simulink model "VelocityControl"  (R2024b)
settings: Solver=VariableStepAuto  StartTime=0.0  StopTime=60  RelTol=1e-3
undefined symbols (not defined in the file or in its folder): Kdu, Kdw, Kiu, Kiw, Kpu, Kpw
libraries: slpidlib x2
settings Model: Creator=Arghya  LastModifiedBy=Arghya

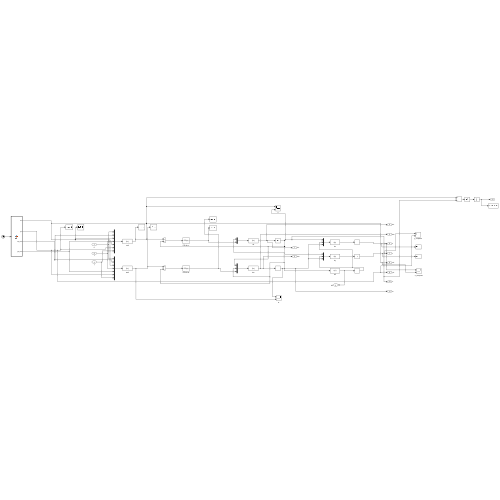
[thumbnail: Simulink's stored preview of the top-level diagram]
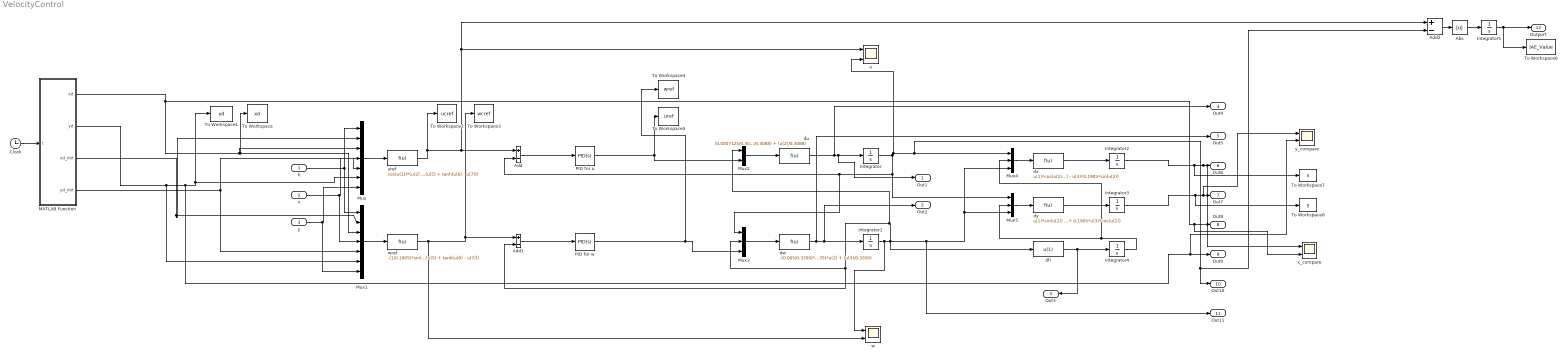
== system VelocityControl ==
  fi : Inport
  x : Inport  Port=2
  y : Inport  Port=3
  Abs : Abs  SaturateOnIntegerOverflow=off
  Add : Sum  Inputs=+-
  Add1 : Sum  Inputs=+-
  Add2 : Sum  Inputs=+-
  Clock : Clock
  Integrator : Integrator  ContinuousStateAttributes="\"u\""
  Integrator1 : Integrator  ContinuousStateAttributes="\"w\""
  Integrator{2..5} (4 alike) : Integrator
  MATLAB Function : MATLAB Function  TreatAsAtomicUnit=on
  Mux : Mux  Inputs=7
  Mux1 : Mux  Inputs=7
  Mux2 : Mux  Inputs=2
  Mux3 : Mux  Inputs=3
  Mux4 : Mux  Inputs=3
  Mux5 : Mux  Inputs=3
  PID for u : slpidlib/PID Controller  Controller=PID  Form=Parallel  TimeDomain=Continuous-time  UseExternalTs=off  SampleTime=-1  IntegratorMethod=Forward Euler  FilterMethod=Forward Euler  ControllerParametersSource=internal  P=Kpu  I=Kiu  UseKiTs=off  D=Kdu  UseExternalDerivativeSource=off  N=100  UseFilter=on  TunerSelectOption=Transfer Function Based (PID Tuner App)  InitialConditionSource=internal  InitialConditionForIntegrator=0  InitialConditionForFilter=0  DifferentiatorICPrevScaledInput=0  ExternalReset=none  TrackingMode=off  Kt=1  LimitOutput=off  SatLimitsSource=internal  UpperSaturationLimit=inf  LowerSaturationLimit=-inf  LinearizeAsGain=on  AntiWindupMode=none  Kb=1  LimitIntegrator=off  UpperIntegratorSaturationLimit=inf  LowerIntegratorSaturationLimit=-inf  POutMin=[]  POutMax=[]  IOutMin=[]  IOutMax=[]  DOutMin=[]  DOutMax=[]  NOutMin=[]  NOutMax=[]  SumOutMin=[]  SumOutMax=[]  SaturationOutMin=[]  SaturationOutMax=[]  PParamMin=[]  PParamMax=[]  IParamMin=[]  IParamMax=[]  DParamMin=[]  DParamMax=[]  NParamMin=[]  NParamMax=[]  KbParamMin=[]  KbParamMax=[]  KtParamMin=[]  KtParamMax=[]  KbOutMin=[]  KbOutMax=[]  KtOutMin=[]  KtOutMax=[]  IntegratorOutMin=[]  IntegratorOutMax=[]  FilterOutMin=[]  FilterOutMax=[]  SumI1OutMin=[]  SumI1OutMax=[]  SumI2OutMin=[]  SumI2OutMax=[]  SumI3OutMin=[]  SumI3OutMax=[]  SumI4OutMin=[]  SumI4OutMax=[]  SumDOutMin=[]  SumDOutMax=[]  DifferentiatorOutMin=[]  DifferentiatorOutMax=[]  FilterDiffOutCoefMin=[]  FilterDiffOutCoefMax=[]  ReciprocalOutMin=[]  ReciprocalOutMax=[]  SumDenOutMin=[]  SumDenOutMax=[]  SumNumOutMin=[]  SumNumOutMax=[]  DivideOutMin=[]  DivideOutMax=[]  UdiffTsProdOutMin=[]  UdiffTsProdOutMax=[]  NTsProdOutMin=[]  NTsProdOutMax=[]  UintegralTsProdOutMin=[]  UintegralTsProdOutMax=[]  UngainTsProdOutMin=[]  UngainTsProdOutMax=[]  ClampingZeroOutDataTypeStr=Inherit: Inherit via back propagation  ClampingZeroOutMin=[]  ClampingZeroOutMax=[]  FilterDenConstantOutDataTypeStr=Inherit: Inherit via back propagation  FilterDenConstantOutMin=[]  FilterDenConstantOutMax=[]  PCopyOutDataTypeStr=Inherit: Inherit via back propagation  PCopyOutMin=[]  PCopyOutMax=[]  NCopyOutDataTypeStr=Inherit: Inherit via back propagation  NCopyOutMin=[]  NCopyOutMax=[]  IntegratorContinuousStateAttributes=''  IntegratorStateMustResolveToSignalObject=off  IntegratorRTWStateStorageClass=Auto  FilterContinuousStateAttributes=''  FilterStateMustResolveToSignalObject=off  FilterRTWStateStorageClass=Auto  ParallelPVariant=InternalParameters  IdealPVariant=Disabled  IVariant=InternalParameters  DVariant=InternalParameters  IntegratorVariant=Continuous  SatVariant=Disabled  AWVariant=Passthrough  PCopyVariant=Disabled  TRVariant=Disabled  FdbkBlocksVariant=Forward  IdealPFdbkVariant=Disabled  SatFdbkVariant=Disabled  DerivativeFilterVariant=ContFilter  NVariant=InternalParameters  NCopyVariant=Disabled  FilterICVariant=InternalICsFilter  IntegratorICVariant=InternalICs  ExternalResetVariant=Disabled  TRSumVariant=Passthrough  SumFdbkVariant=Disabled  SumVariant=Sum_PID  TsampFilterVariant=InternalTs  TsampNgainVariant=Passthrough  TsampIntegralVariant=Disabled_SignalSpec  ExternalSaturationOutDataTypeStr=Inherit: Same as second input  DerivativeSourceVariant=ErrorSignal  PreIntVariant=InternalPreInt
  PID for w : slpidlib/PID Controller  Controller=PID  Form=Parallel  TimeDomain=Continuous-time  UseExternalTs=off  SampleTime=-1  IntegratorMethod=Forward Euler  FilterMethod=Forward Euler  ControllerParametersSource=internal  P=Kpw  I=Kiw  UseKiTs=off  D=Kdw  UseExternalDerivativeSource=off  N=100  UseFilter=on  TunerSelectOption=Transfer Function Based (PID Tuner App)  InitialConditionSource=internal  InitialConditionForIntegrator=0  InitialConditionForFilter=0  DifferentiatorICPrevScaledInput=0  ExternalReset=none  TrackingMode=off  Kt=1  LimitOutput=off  SatLimitsSource=internal  UpperSaturationLimit=inf  LowerSaturationLimit=-inf  LinearizeAsGain=on  AntiWindupMode=none  Kb=1  LimitIntegrator=off  UpperIntegratorSaturationLimit=inf  LowerIntegratorSaturationLimit=-inf  POutMin=[]  POutMax=[]  IOutMin=[]  IOutMax=[]  DOutMin=[]  DOutMax=[]  NOutMin=[]  NOutMax=[]  SumOutMin=[]  SumOutMax=[]  SaturationOutMin=[]  SaturationOutMax=[]  PParamMin=[]  PParamMax=[]  IParamMin=[]  IParamMax=[]  DParamMin=[]  DParamMax=[]  NParamMin=[]  NParamMax=[]  KbParamMin=[]  KbParamMax=[]  KtParamMin=[]  KtParamMax=[]  KbOutMin=[]  KbOutMax=[]  KtOutMin=[]  KtOutMax=[]  IntegratorOutMin=[]  IntegratorOutMax=[]  FilterOutMin=[]  FilterOutMax=[]  SumI1OutMin=[]  SumI1OutMax=[]  SumI2OutMin=[]  SumI2OutMax=[]  SumI3OutMin=[]  SumI3OutMax=[]  SumI4OutMin=[]  SumI4OutMax=[]  SumDOutMin=[]  SumDOutMax=[]  DifferentiatorOutMin=[]  DifferentiatorOutMax=[]  FilterDiffOutCoefMin=[]  FilterDiffOutCoefMax=[]  ReciprocalOutMin=[]  ReciprocalOutMax=[]  SumDenOutMin=[]  SumDenOutMax=[]  SumNumOutMin=[]  SumNumOutMax=[]  DivideOutMin=[]  DivideOutMax=[]  UdiffTsProdOutMin=[]  UdiffTsProdOutMax=[]  NTsProdOutMin=[]  NTsProdOutMax=[]  UintegralTsProdOutMin=[]  UintegralTsProdOutMax=[]  UngainTsProdOutMin=[]  UngainTsProdOutMax=[]  ClampingZeroOutDataTypeStr=Inherit: Inherit via back propagation  ClampingZeroOutMin=[]  ClampingZeroOutMax=[]  FilterDenConstantOutDataTypeStr=Inherit: Inherit via back propagation  FilterDenConstantOutMin=[]  FilterDenConstantOutMax=[]  PCopyOutDataTypeStr=Inherit: Inherit via back propagation  PCopyOutMin=[]  PCopyOutMax=[]  NCopyOutDataTypeStr=Inherit: Inherit via back propagation  NCopyOutMin=[]  NCopyOutMax=[]  IntegratorContinuousStateAttributes=''  IntegratorStateMustResolveToSignalObject=off  IntegratorRTWStateStorageClass=Auto  FilterContinuousStateAttributes=''  FilterStateMustResolveToSignalObject=off  FilterRTWStateStorageClass=Auto  ParallelPVariant=InternalParameters  IdealPVariant=Disabled  IVariant=InternalParameters  DVariant=InternalParameters  IntegratorVariant=Continuous  SatVariant=Disabled  AWVariant=Passthrough  PCopyVariant=Disabled  TRVariant=Disabled  FdbkBlocksVariant=Forward  IdealPFdbkVariant=Disabled  SatFdbkVariant=Disabled  DerivativeFilterVariant=ContFilter  NVariant=InternalParameters  NCopyVariant=Disabled  FilterICVariant=InternalICsFilter  IntegratorICVariant=InternalICs  ExternalResetVariant=Disabled  TRSumVariant=Passthrough  SumFdbkVariant=Disabled  SumVariant=Sum_PID  TsampFilterVariant=InternalTs  TsampNgainVariant=Passthrough  TsampIntegralVariant=Disabled_SignalSpec  ExternalSaturationOutDataTypeStr=Inherit: Same as second input  DerivativeSourceVariant=ErrorSignal  PreIntVariant=InternalPreInt
  To Workspace : ToWorkspace  VariableName=xd  SampleTime=-1
  To Workspace1 : ToWorkspace  VariableName=yd  SampleTime=-1
  To Workspace2 : ToWorkspace  VariableName=ucref  SaveFormat=Timeseries  SampleTime=-1
  To Workspace3 : ToWorkspace  VariableName=wcref  SaveFormat=Timeseries  SampleTime=-1
  To Workspace4 : ToWorkspace  VariableName=wref  SaveFormat=Timeseries  SampleTime=-1
  To Workspace5 : ToWorkspace  VariableName=uref  SaveFormat=Timeseries  SampleTime=-1
  To Workspace6 : ToWorkspace  VariableName=IAE_Value  SampleTime=-1
  To Workspace7 : ToWorkspace  VariableName=x  SampleTime=-1
  To Workspace8 : ToWorkspace  VariableName=y  SampleTime=-1
  dfi : Fcn  Expr=u(1)
  du : Fcn  Expr=(0.0007125/0.3088)*u(1)*u(1) - (1.2484/0.3088) + (u(2)/0.3088)
  dw : Fcn  Expr=-(0.005/0.3350)*u(1)*u(2) - (1.3207/0.335)*u(2) + (u(3)/0.3350)
  dx : Fcn  Expr=u(1)*cos(u(2)) - u(3)*0.1905*sin(u(2))
  dy : Fcn  Expr=u(1)*sin(u(2)) + 0.1905*u(3)*cos(u(2))
  u : Scope  NumInputPorts=2
  uref : Fcn  Expr=cos(u(1))*(u(2) + tanh(u(3) - u(4))) + sin(u(1))*(u(5) + tanh(u(6) - u(7)))
  w : Scope  NumInputPorts=2
  wref : Fcn  Expr=-(1/0.1905)*sin(u(1))*(u(2) + tanh(u(3) - u(4))) + (1/0.1905)*cos(u(1))*(u(5) + tanh(u(6) - u(7)))
  x_compare : Scope  NumInputPorts=2
  y_compare : Scope  NumInputPorts=2
  Out1 : Outport  SignalName=du
  Out2 : Outport  Port=2  SignalName=dw
  Out3 : Outport  Port=3  SignalName=dfi
  Out4 : Outport  Port=4  SignalName=du
  Out5 : Outport  Port=5  SignalName=dw
  Out6 : Outport  Port=6  SignalName=x
  Out7 : Outport  Port=7  SignalName=y
  Out8 : Outport  Port=8  SignalName=xd
  Out9 : Outport  Port=9  SignalName=yd
  Out10 : Outport  Port=10  SignalName=u
  Out11 : Outport  Port=11  SignalName=w
  Outport : Outport  Port=12
  wires:
  MATLAB Function/2(yd) -> Mux1/6, y_compare/2, Out9/1, Mux/6, To Workspace1/1
  MATLAB Function/1(xd) -> Mux1/3, To Workspace/1, Mux/3, x_compare/2, Out8/1
  fi/1 -> Mux1/1, Mux/1
  MATLAB Function/3(xd_dot) -> Mux/2, Mux1/2
  x/1 -> Mux1/4, Mux/4
  MATLAB Function/4(yd_dot) -> Mux1/5, Mux/5
  y/1 -> Mux1/7, Mux/7
  Mux/1 -> uref/1
  Mux1/1 -> wref/1
  wref/1 -> w/2, To Workspace3/1, Add1/1
  Add/1 -> PID for u/1
  Add1/1 -> PID for w/1
  Mux3/1 -> dw/1
  Mux2/1 -> du/1
  du/1 -> Out4/1, Out1/1, Integrator/1
  dw/1 -> Out5/1, Out2/1, Integrator1/1
  Integrator1/1 -> w/1, dfi/1, Out11/1, Mux5/3, Mux4/3, Mux2/1, Add1/2, Mux3/2
  Integrator/1 -> u/2, Add2/2, Out10/1, Mux4/1, Mux5/1, Add/2, Mux3/1
  PID for u/1 -> Mux2/2, To Workspace5/1
  PID for w/1 -> Mux3/3, To Workspace4/1
  Mux4/1 -> dx/1
  Mux5/1 -> dy/1
  dfi/1 -> Out3/1, Integrator4/1
  dy/1 -> Integrator3/1
  dx/1 -> Integrator2/1
  Integrator4/1 -> Mux5/2, Mux4/2
  Integrator2/1 -> To Workspace7/1, x_compare/1, Out6/1
  Integrator3/1 -> To Workspace8/1, y_compare/1, Out7/1
  Clock/1 -> MATLAB Function/1(t)
  uref/1 -> u/1, Add2/1, Add/1, To Workspace2/1
  Add2/1 -> Abs/1
  Abs/1 -> Integrator5/1
  Integrator5/1 -> To Workspace6/1, Outport/1

== matlab function VelocityControl/MATLAB Function ==
  data: t input; xd output; yd output; xd_dot output; yd_dot output
function [xd, yd, xd_dot, yd_dot] = fcn(t)

% Define trajectory parameters. Adjust these values to change the size and shape.
A = 1.0;
B = 1.0;
w1 = 1.0;
w2 = 1.0;

% Calculate desired positions (8-shape)
xd = A * sin(w1 * t);
yd = B * sin(w2 * t) * cos(w1 * t);

% Calculate desired velocities (first derivative of positions)
xd_dot = A * w1 * cos(w1 * t);
yd_dot = B * w2 * cos(w2 * t) * cos(w1 * t) - B * w1 * sin(w2 * t) * sin(w1 * t);

end
